simulink model "kinematics_model"  (R2023a)
settings: Solver=FixedStepAuto  StartTime=0.0  StopTime=fs  FixedStep=ts  RelTol=1e-3
undefined symbols (not defined in the file): alpha, eta_0, K_p, k_R, k_theta, p_0, theta_d, umax, umin, y_d
libraries: simulink_extras x1, slctrlblks x1, simulink x1
settings Model: Creator=mori_keigo  LastModifiedBy=mori_keigo

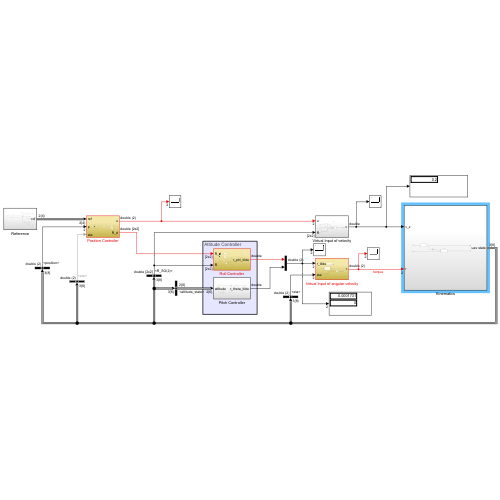
[thumbnail: Simulink's stored preview of the top-level diagram]
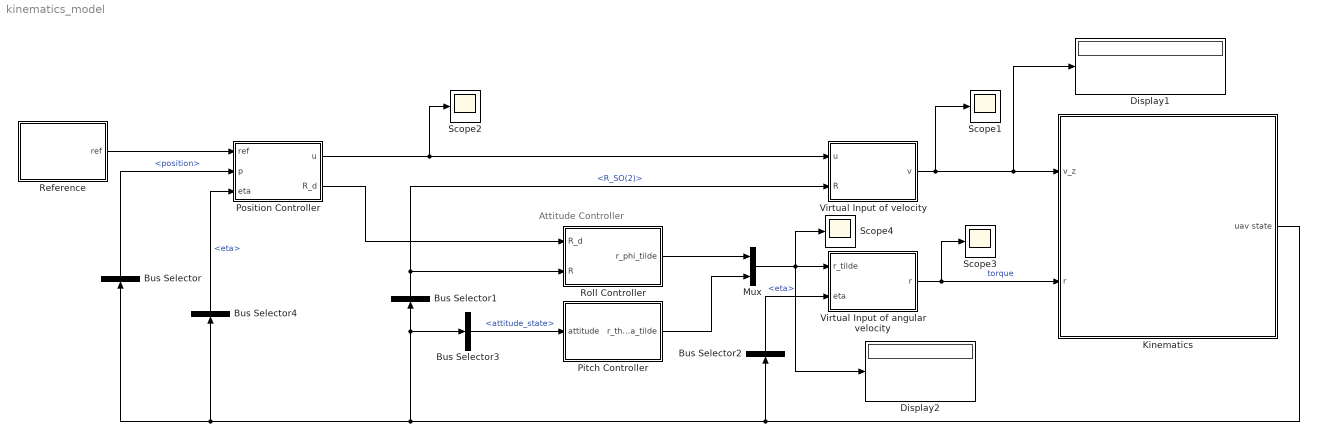
== system kinematics_model ==
  note: Attitude Controller
  Bus Selector : BusSelector  OutputSignals=translation_state.position
  Bus Selector1 : BusSelector  OutputSignals=attitude_state.R_SO(2)
  Bus Selector2 : BusSelector  OutputSignals=attitude_state.eta
  Bus Selector3 : BusSelector  OutputSignals=attitude_state
  Bus Selector4 : BusSelector  OutputSignals=attitude_state.eta
  Display1 : Display
  Display2 : Display
  Kinematics : Subsystem
  Mux : Mux  Inputs=2
  Pitch Controller : Subsystem
  Position Controller : Subsystem
  Reference : Subsystem
  Roll Controller : Subsystem
  Scope{1..4} (4 alike) : Scope
  Virtual Input of angular velocity : Subsystem
  Virtual Input of velocity : Subsystem
  wires:
  Bus Selector/1 -> Position Controller/2(p)  "<position>"
  Reference/1(ref) -> Position Controller/1(ref)
  Position Controller/2(R_d) -> Roll Controller/1(R_d)
  Kinematics/1(uav state) -> Bus Selector/1, Bus Selector4/1, Bus Selector1/1, Bus Selector3/1, Bus Selector2/1
  Virtual Input of velocity/1(v) -> Display1/1, Kinematics/1(v_z), Scope1/1
  Roll Controller/1(r_phi_tilde) -> Mux/1
  Pitch Controller/1(r_theta_tilde) -> Mux/2
  Mux/1 -> Scope4/1, Display2/1, Virtual Input of angular velocity/1(r_tilde)
  Bus Selector3/1 -> Pitch Controller/1(attitude)  "<attitude_state>"
  Bus Selector1/1 -> Roll Controller/2(R), Virtual Input of velocity/2(R)  "<R_SO(2)>"
  Bus Selector2/1 -> Virtual Input of angular velocity/2(eta)  "<eta>"
  Position Controller/1(u) -> Scope2/1, Virtual Input of velocity/1(u)
  Bus Selector4/1 -> Position Controller/3(eta)  "<eta>"
  Virtual Input of angular velocity/1(r) -> Kinematics/2(r), Scope3/1  "torque"

== system kinematics_model/Kinematics ==
  note: $\dot{\eta} = A r$
  note: $\dot{p} = Rv$
  v_z : Inport
  r : Inport  Port=2
  Bus Selector : BusSelector  OutputSignals=eta
  Kinematics of Attitude : Subsystem
  Kinematics of Translation : Subsystem
  Out Bus Element : Outport  PortName=uav state  Element=attitude_state
  Out Bus Element1 : Outport  PortName=uav state  Element=translation_state
  wires:
  r/1 -> Kinematics of Attitude/1(r)
  Kinematics of Translation/1(uav state) -> Out Bus Element1/1  "translation_state"
  v_z/1 -> Kinematics of Translation/2(v_z)  "attitude_state"
  Kinematics of Attitude/1(attitude_state) -> Bus Selector/1, Out Bus Element/1
  Bus Selector/1 -> Kinematics of Translation/1(eta)  "<eta>"

== system kinematics_model/Pitch Controller ==
  note: $\tilde{r}_{\theta} = k_{\theta} (\theta_d - \theta)$
  attitude : Inport
  Bus Selector : BusSelector  OutputSignals=eta
  Gain : Gain  Gain=k_theta
  Selector : Selector  InputPortWidth=2  IndexOptions=Index vector (dialog)  Indices=[2]  OutputSizes=1
  Sum : Sum  Inputs=|+-
  theta_d : Constant  Value=theta_d
  r_theta_tilde : Outport
  wires:
  attitude/1 -> Bus Selector/1
  theta_d/1 -> Sum/1
  Sum/1 -> Gain/1
  Gain/1 -> r_theta_tilde/1
  Bus Selector/1 -> Selector/1  "<eta>"
  Selector/1 -> Sum/2

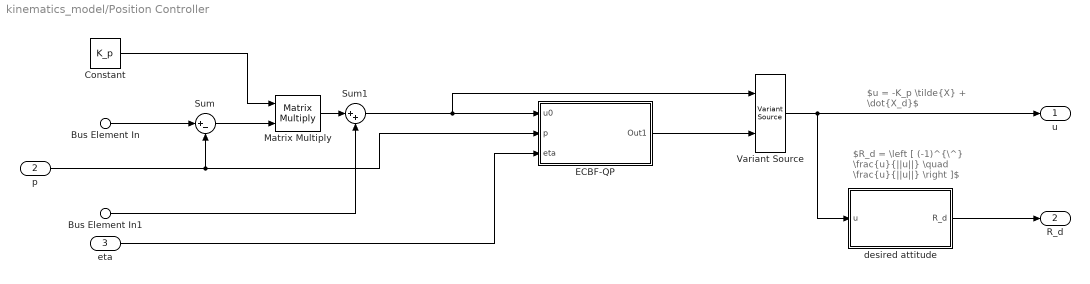
== system kinematics_model/Position Controller ==
  note: $u = -K_p \tilde{X} + \dot{X_d}$
  note: $R_d = \left [ (-1)^{\^} \frac{u}{||u||} \quad \frac{u}{||u||} \right ]$
  Bus Element In : Inport  PortName=ref  Element=p_d
  Bus Element In1 : Inport  PortName=ref  Element=p_d_dot
  p : Inport  Port=2
  eta : Inport  Port=3
  Constant : Constant  Value=K_p
  ECBF-QP : Subsystem
  Matrix Multiply : Product  Multiplication=Matrix(*)
  Sum : Sum  Inputs=|+-
  Sum1 : Sum  Inputs=|++
  Variant Source : VariantSource
  desired attitude : Subsystem
  u : Outport
  R_d : Outport  Port=2
  wires:
  Bus Element In/1 -> Sum/1
  Bus Element In1/1 -> Sum1/2
  desired attitude/1(R_d) -> R_d/1
  Matrix Multiply/1 -> Sum1/1
  Constant/1 -> Matrix Multiply/1
  Sum/1 -> Matrix Multiply/2
  Sum1/1 -> Variant Source/1, ECBF-QP/1(u0)
  ECBF-QP/1(Out1) -> Variant Source/2
  eta/1 -> ECBF-QP/3(eta)
  Variant Source/1 -> desired attitude/1(u), u/1
  p/1 -> ECBF-QP/2(p), Sum/2

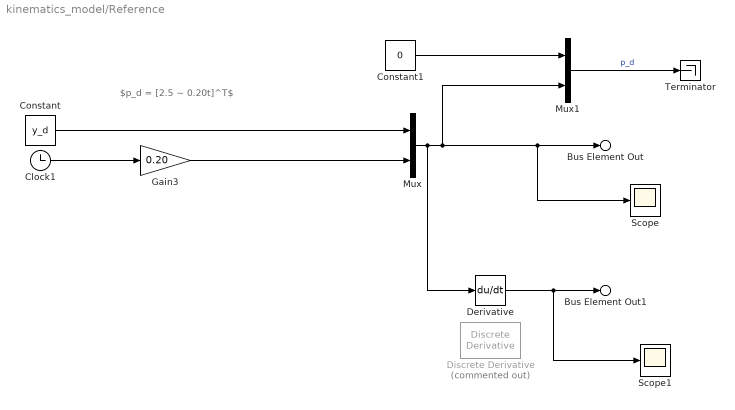
== system kinematics_model/Reference ==
  note: $p_d = [2.5 ~ 0.20t]^T$
  Clock1 : Clock
  Constant : Constant  Value=y_d
  Constant1 : Constant  Value=0
  Derivative : Derivative
  Discrete Derivative : simulink/Discrete/Discrete Derivative  Commented=on  gainval=1.0  ICPrevScaledInput=0.0  OutMin=[]  OutMax=[]  OutDataType=fixdt(1, 16)  OutScaling=2^-10  DoSatur=off
  Gain3 : Gain  Gain=0.20
  Mux : Mux  Inputs=2
  Mux1 : Mux  Inputs=2
  Scope : Scope
  Scope1 : Scope
  Terminator : Terminator
  Bus Element Out : Outport  PortName=ref  Element=p_d
  Bus Element Out1 : Outport  PortName=ref  Element=p_d_dot
  wires:
  Derivative/1 -> Scope1/1, Bus Element Out1/1
  Clock1/1 -> Gain3/1
  Gain3/1 -> Mux/2
  Mux/1 -> Mux1/2, Scope/1, Bus Element Out/1, Derivative/1
  Constant1/1 -> Mux1/1
  Mux1/1 -> Terminator/1  "p_d"
  Constant/1 -> Mux/1

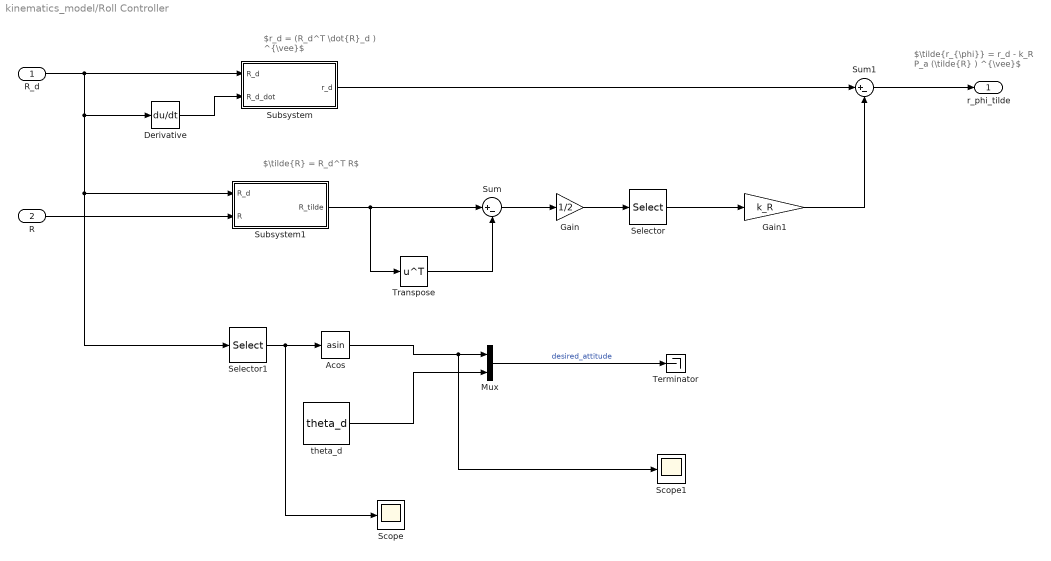
== system kinematics_model/Roll Controller ==
  note: $r_d = (R_d^T \dot{R}_d ) ^{\vee}$
  note: $\tilde{r_{\phi}} = r_d - k_R P_a (\tilde{R} ) ^{\vee}$
  note: $\tilde{R} = R_d^T R$
  R_d : Inport
  R : Inport  Port=2
  Acos : Trigonometry  Operator=asin
  Derivative : Derivative
  Gain : Gain  Gain=1/2
  Gain1 : Gain  Gain=k_R
  Mux : Mux  Inputs=2
  Scope : Scope
  Scope1 : Scope
  Selector : Selector  NumberOfDimensions=2  InputPortWidth=3  IndexOptions=Index vector (dialog),Index vector (dialog)  Indices=[2],1  OutputSizes=1,1
  Selector1 : Selector  NumberOfDimensions=2  InputPortWidth=3  IndexOptions=Index vector (dialog),Index vector (dialog)  Indices=[2],[1]  OutputSizes=1,1
  Subsystem : Subsystem
  Subsystem1 : Subsystem
  Sum : Sum  Inputs=|+-
  Sum1 : Sum  Inputs=|+-
  Terminator : Terminator
  Transpose : Math  Operator=transpose
  theta_d : Constant  Value=theta_d
  r_phi_tilde : Outport
  wires:
  Derivative/1 -> Subsystem/2(R_d_dot)
  Subsystem1/1(R_tilde) -> Transpose/1, Sum/1
  Transpose/1 -> Sum/2
  Sum/1 -> Gain/1
  Gain/1 -> Selector/1
  Selector/1 -> Gain1/1
  Sum1/1 -> r_phi_tilde/1
  Subsystem/1(r_d) -> Sum1/1
  Gain1/1 -> Sum1/2
  R_d/1 -> Selector1/1, Subsystem1/1(R_d), Derivative/1, Subsystem/1(R_d)
  Selector1/1 -> Scope/1, Acos/1
  R/1 -> Subsystem1/2(R)
  Acos/1 -> Scope1/1, Mux/1
  theta_d/1 -> Mux/2
  Mux/1 -> Terminator/1  "desired_attitude"

== system kinematics_model/Virtual Input of angular velocity ==
  note: $r = A^{-1} \tilde{r}$
  r_tilde : Inport
  eta : Inport  Port=2
  Product : Product  Inputs=/*  Multiplication=Matrix(*)
  Transformation to A : Subsystem
  r : Outport
  wires:
  Transformation to A/1(A) -> Product/1
  r_tilde/1 -> Product/2
  Product/1 -> r/1
  eta/1 -> Transformation to A/1(eta)

== system kinematics_model/Virtual Input of velocity ==
  note: $v_z = u^T Re_2$
  u : Inport
  R : Inport  Port=2
  Constant : Constant  Value=[0;1]  VectorParams1D=off
  Matrix Multiply : Product  Inputs=3  Multiplication=Matrix(*)
  Transpose : Math  Operator=transpose
  v : Outport
  wires:
  R/1 -> Matrix Multiply/2
  Transpose/1 -> Matrix Multiply/1
  Matrix Multiply/1 -> v/1
  u/1 -> Transpose/1
  Constant/1 -> Matrix Multiply/3

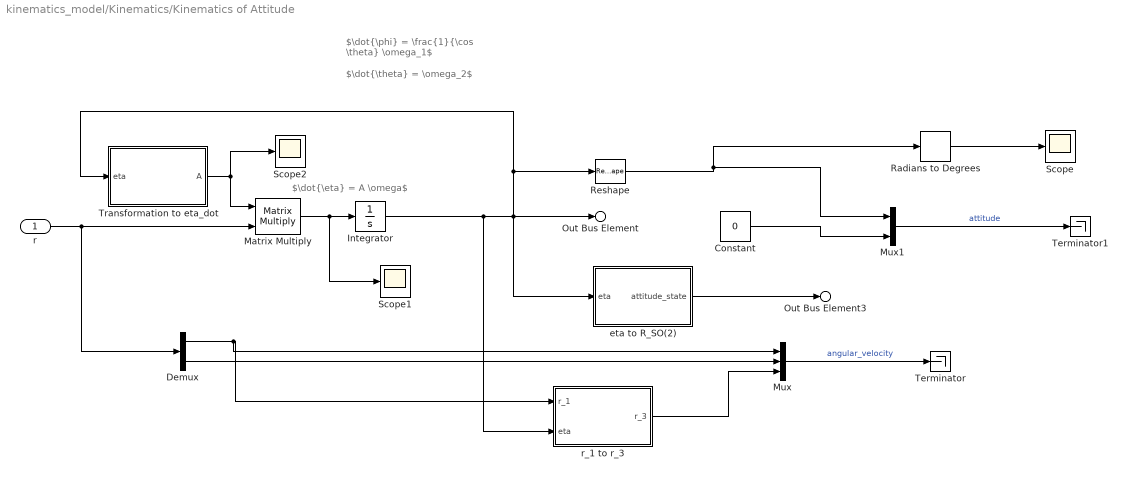
== system kinematics_model/Kinematics/Kinematics of Attitude ==
  note: $\dot{\theta} = \omega_2$
  note: $\dot{\phi} = \frac{1}{\cos \theta} \omega_1$
  note: $\dot{\eta} = A \omega$
  r : Inport
  Constant : Constant  Value=0
  Demux : Demux  Outputs=2
  Integrator : Integrator  InitialCondition=eta_0
  Matrix Multiply : Product  Multiplication=Matrix(*)
  Mux : Mux  Inputs=3
  Mux1 : Mux  Inputs=2
  Radians to Degrees : simulink_extras/Transformations/Radians to Degrees
  Reshape : Reshape
  Scope : Scope
  Scope1 : Scope
  Scope2 : Scope
  Terminator : Terminator
  Terminator1 : Terminator
  Transformation to eta_dot : Subsystem
  eta to R_SO(2) : Subsystem
  r_1 to r_3 : Subsystem
  Out Bus Element : Outport  PortName=attitude_state  Element=eta
  Out Bus Element3 : Outport  PortName=attitude_state  Element=R_SO(2)
  wires:
  Integrator/1 -> r_1 to r_3/2(eta), Out Bus Element/1, eta to R_SO(2)/1(eta), Transformation to eta_dot/1(eta), Reshape/1
  Matrix Multiply/1 -> Scope1/1, Integrator/1
  r/1 -> Demux/1, Matrix Multiply/2
  Transformation to eta_dot/1(A) -> Matrix Multiply/1, Scope2/1
  eta to R_SO(2)/1(attitude_state) -> Out Bus Element3/1
  Demux/1 -> Mux/1, r_1 to r_3/1(r_1)
  r_1 to r_3/1(r_3) -> Mux/3
  Demux/2 -> Mux/2
  Mux/1 -> Terminator/1  "angular_velocity"
  Radians to Degrees/1 -> Scope/1
  Reshape/1 -> Mux1/1, Radians to Degrees/1
  Constant/1 -> Mux1/2
  Mux1/1 -> Terminator1/1  "attitude"

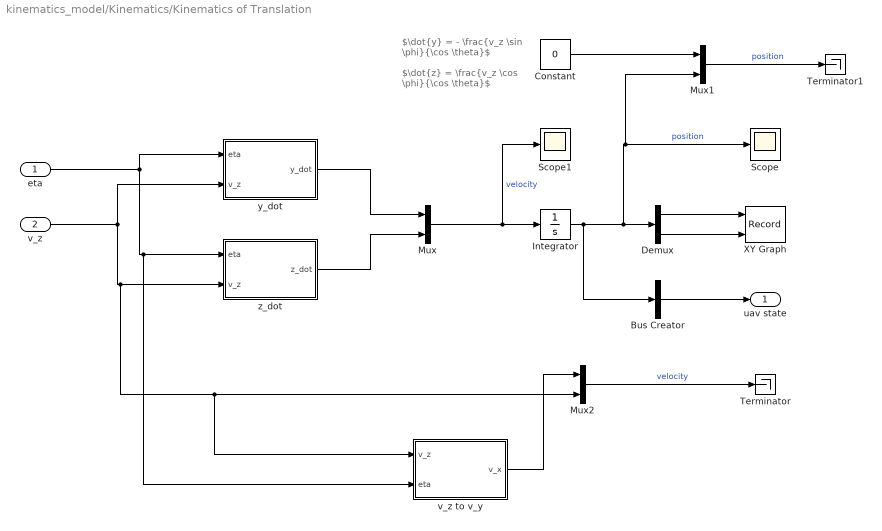
== system kinematics_model/Kinematics/Kinematics of Translation ==
  note: $\dot{z} = \frac{v_z \cos \phi}{\cos \theta}$
  note: $\dot{y} = - \frac{v_z \sin \phi}{\cos \theta}$
  eta : Inport
  v_z : Inport  Port=2
  Bus Creator : BusCreator  Inputs=1
  Constant : Constant  Value=0
  Demux : Demux  Outputs=2
  Integrator : Integrator  InitialCondition=p_0
  Mux : Mux  Inputs=2
  Mux1 : Mux  Inputs=2
  Mux2 : Mux  Inputs=2
  Scope : Scope
  Scope1 : Scope
  Terminator : Terminator
  Terminator1 : Terminator
  XY Graph : Record  FileSettingsInternal="{\"entries\":[{\"content\":{\"excelSettings\":{\"content\":{},\"type\":\"Streamout.ExcelSettings\"}},\"type\":\"Streamout.FileSettingStorage\",\"uuid\":\"\"}],\"packageUris\":[\"http:\\/\\/schema.mathworks.com\\/mf0\\/streamout_blocks\\/R2020a\"],\"version\":\"1.0\"}"  Layout=[1 1]  SignalsInternal="{\"entries\":[{\"content\":{\"signals\":[{\"content\":{\"blockPath\":[],\"dimensions\":[1],\"domain\":\"\",\"lineColor\":\"#a2142f\",\"plots\":[1],\"port\":1,\"sid\":[\"\"],\"signalID\":39,\"signalName\":\"Demux:1\"},\"type\":\"RecordBlkView.Signal\",\"uuid\":\"\"},{\"content\":{\"blockPath\":[],\"dimensions\":[1],\"domain\":\"\",\"lineColor\":\"#139fff\",\"plots\":[1],\"port\":2,\"sid\":[\"\"],\"signalID\":43,\"signalName\":\"Demux:2\"},\"type\":\"RecordBlkView.Signal\",\"uuid\":\"\"}]},\"type\":\"RecordBlkView.InputSignals\",\"uuid\":\"\"}],\"packageUris\":[\"http:\\/\\/schema.mathworks.com\\/mf0\\/streamout_blocks\\/R2020a\"],\"version\":\"1.0\"}"  VisualizationBindings="{\"xyplotplugin\":{\"info\":[{\"series\":[{\"bindingParametersList\":[{\"parameter\":\"X-Axis\",\"signalID\":39,\"signalName\":\"Demux:1\"},{\"parameter\":\"Y-Axis\",\"signalID\":43,\"signalName\":\"Demux:2\"}],\"seriesID\":24023}],\"subplotID\":1}]}}"  CompatibilityTag=XY
  v_z to v_y : Subsystem
  y_dot : Subsystem
  z_dot : Subsystem
  uav state : Outport
  wires:
  Integrator/1 -> Mux1/2, Scope/1, Demux/1, Bus Creator/1  "position"
  Mux/1 -> Scope1/1, Integrator/1  "velocity"
  Bus Creator/1 -> uav state/1
  eta/1 -> v_z to v_y/2(eta), z_dot/1(eta), y_dot/1(eta)
  y_dot/1(y_dot) -> Mux/1
  v_z/1 -> v_z to v_y/1(v_z), Mux2/2, z_dot/2(v_z), y_dot/2(v_z)
  z_dot/1(z_dot) -> Mux/2
  Demux/1 -> XY Graph/1
  Demux/2 -> XY Graph/2
  Mux2/1 -> Terminator/1  "velocity"
  v_z to v_y/1(v_x) -> Mux2/1
  Constant/1 -> Mux1/1
  Mux1/1 -> Terminator1/1  "position"

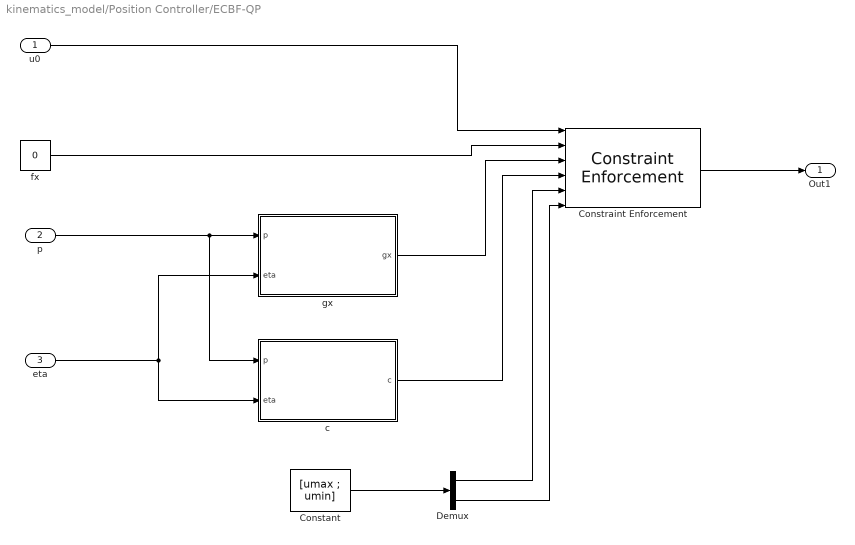
== system kinematics_model/Position Controller/ECBF-QP ==
  u0 : Inport
  p : Inport  Port=2
  eta : Inport  Port=3
  Constant : Constant  Value=[umax ; umin]  VectorParams1D=off
  Constraint Enforcement : slctrlblks/Constraint Enforcement  nc=1  nu=2  c=0  external_c=on  external_umax=on  external_umin=on  Ts=0.01  maxiter=200  tol=1e-6  output_exitflag=off  relax_c=off  relax_u=off
  Demux : Demux  Outputs=2
  c : Subsystem
  fx : Constant  Value=0  VectorParams1D=off
  gx : Subsystem
  Out1 : Outport
  wires:
  u0/1 -> Constraint Enforcement/1
  p/1 -> c/1(p), gx/1(p)
  eta/1 -> gx/2(eta), c/2(eta)
  fx/1 -> Constraint Enforcement/2
  gx/1(gx) -> Constraint Enforcement/3
  c/1(c) -> Constraint Enforcement/4
  Constraint Enforcement/1 -> Out1/1
  Constant/1 -> Demux/1
  Demux/1 -> Constraint Enforcement/5
  Demux/2 -> Constraint Enforcement/6

== system kinematics_model/Position Controller/desired attitude ==
  u : Inport
  (-1)^ : Constant  Value=[0 1; -1 0]  VectorParams1D=off
  Divide : Product  Inputs=*/
  Dot Product : DotProduct  OutDataTypeStr=Inherit: Inherit via internal rule
  Matrix Concatenate : Concatenate  Mode=Multidimensional array  ConcatenateDimension=2
  Matrix Multiply : Product  Multiplication=Matrix(*)
  Square Root : Sqrt
  R_d : Outport
  wires:
  Dot Product/1 -> Square Root/1
  u/1 -> Divide/1, Dot Product/2, Dot Product/1
  Square Root/1 -> Divide/2
  Matrix Concatenate/1 -> R_d/1
  Divide/1 -> Matrix Concatenate/2, Matrix Multiply/2
  (-1)^/1 -> Matrix Multiply/1
  Matrix Multiply/1 -> Matrix Concatenate/1

== system kinematics_model/Roll Controller/Subsystem ==
  R_d : Inport
  R_d_dot : Inport  Port=2
  Matrix Multiply : Product  Multiplication=Matrix(*)
  Selector : Selector  NumberOfDimensions=2  InputPortWidth=3  IndexOptions=Index vector (dialog),Index vector (dialog)  Indices=[2],1  OutputSizes=1,1
  Transpose : Math  Operator=transpose
  r_d : Outport
  wires:
  R_d/1 -> Transpose/1
  Transpose/1 -> Matrix Multiply/1
  R_d_dot/1 -> Matrix Multiply/2
  Matrix Multiply/1 -> Selector/1
  Selector/1 -> r_d/1

== system kinematics_model/Roll Controller/Subsystem1 ==
  R_d : Inport
  R : Inport  Port=2
  Matrix Multiply : Product  Multiplication=Matrix(*)
  Transpose : Math  Operator=transpose
  R_tilde : Outport
  wires:
  R_d/1 -> Transpose/1
  Transpose/1 -> Matrix Multiply/1
  R/1 -> Matrix Multiply/2
  Matrix Multiply/1 -> R_tilde/1

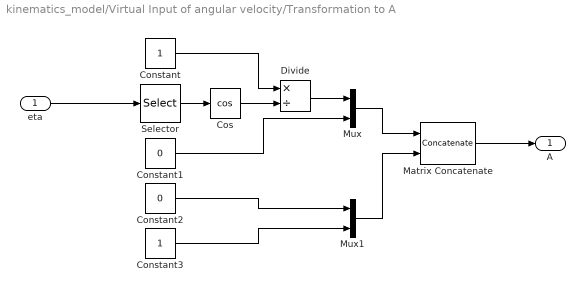
== system kinematics_model/Virtual Input of angular velocity/Transformation to A ==
  eta : Inport
  Constant : Constant
  Constant1 : Constant  Value=0
  Constant2 : Constant  Value=0
  Constant3 : Constant
  Cos : Trigonometry  Operator=cos
  Divide : Product  Inputs=*/
  Matrix Concatenate : Concatenate  Mode=Multidimensional array  ConcatenateDimension=2
  Mux : Mux  Inputs=2
  Mux1 : Mux  Inputs=2
  Selector : Selector  InputPortWidth=2  IndexOptions=Index vector (dialog)  Indices=[2]  OutputSizes=1
  A : Outport
  wires:
  eta/1 -> Selector/1
  Constant/1 -> Divide/1
  Divide/1 -> Mux/1
  Constant1/1 -> Mux/2
  Constant2/1 -> Mux1/1
  Constant3/1 -> Mux1/2
  Mux/1 -> Matrix Concatenate/1
  Mux1/1 -> Matrix Concatenate/2
  Matrix Concatenate/1 -> A/1
  Selector/1 -> Cos/1
  Cos/1 -> Divide/2

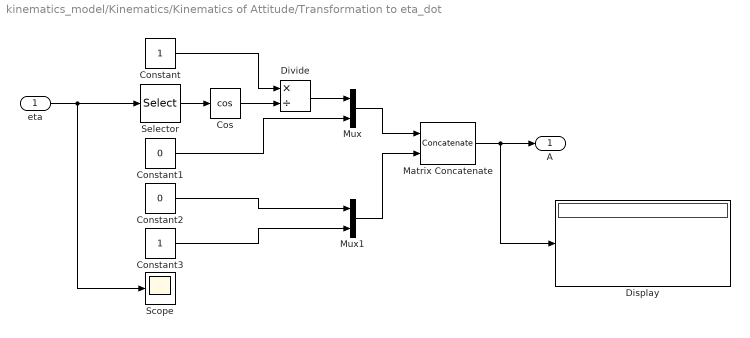
== system kinematics_model/Kinematics/Kinematics of Attitude/Transformation to eta_dot ==
  eta : Inport
  Constant : Constant
  Constant1 : Constant  Value=0
  Constant2 : Constant  Value=0
  Constant3 : Constant
  Cos : Trigonometry  Operator=cos
  Display : Display
  Divide : Product  Inputs=*/
  Matrix Concatenate : Concatenate  Mode=Multidimensional array  ConcatenateDimension=2
  Mux : Mux  Inputs=2
  Mux1 : Mux  Inputs=2
  Scope : Scope
  Selector : Selector  InputPortWidth=2  IndexOptions=Index vector (dialog)  Indices=[2]  OutputSizes=1
  A : Outport
  wires:
  eta/1 -> Scope/1, Selector/1
  Constant/1 -> Divide/1
  Divide/1 -> Mux/1
  Constant1/1 -> Mux/2
  Constant2/1 -> Mux1/1
  Constant3/1 -> Mux1/2
  Mux/1 -> Matrix Concatenate/1
  Mux1/1 -> Matrix Concatenate/2
  Matrix Concatenate/1 -> Display/1, A/1
  Selector/1 -> Cos/1
  Cos/1 -> Divide/2

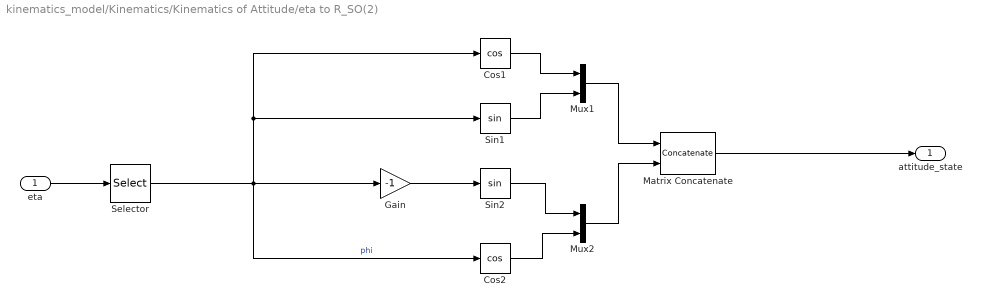
== system kinematics_model/Kinematics/Kinematics of Attitude/eta to R_SO(2) ==
  eta : Inport
  Cos1 : Trigonometry  Operator=cos
  Cos2 : Trigonometry  Operator=cos
  Gain : Gain  Gain=-1
  Matrix Concatenate : Concatenate  Mode=Multidimensional array  ConcatenateDimension=2
  Mux1 : Mux  Inputs=2
  Mux2 : Mux  Inputs=2
  Selector : Selector  InputPortWidth=2  IndexOptions=Index vector (dialog)  Indices=[1]  OutputSizes=1
  Sin1 : Trigonometry
  Sin2 : Trigonometry
  attitude_state : Outport
  wires:
  eta/1 -> Selector/1
  Cos2/1 -> Mux2/2
  Matrix Concatenate/1 -> attitude_state/1
  Mux2/1 -> Matrix Concatenate/2
  Mux1/1 -> Matrix Concatenate/1
  Gain/1 -> Sin2/1
  Cos1/1 -> Mux1/1
  Sin2/1 -> Mux2/1
  Sin1/1 -> Mux1/2
  Selector/1 -> Cos2/1, Gain/1, Cos1/1, Sin1/1  "phi"

== system kinematics_model/Kinematics/Kinematics of Attitude/r_1 to r_3 ==
  r_1 : Inport
  eta : Inport  Port=2
  Cos : Trigonometry  Operator=cos
  Divide : Product  Inputs=**/
  Gain : Gain  Gain=-1
  Selector : Selector  InputPortWidth=2  IndexOptions=Index vector (dialog)  Indices=[2]  OutputSizes=1
  Sin : Trigonometry
  r_3 : Outport
  wires:
  eta/1 -> Selector/1
  Selector/1 -> Cos/1, Sin/1
  r_1/1 -> Divide/1
  Sin/1 -> Divide/2
  Cos/1 -> Divide/3
  Divide/1 -> Gain/1
  Gain/1 -> r_3/1

== system kinematics_model/Kinematics/Kinematics of Translation/v_z to v_y ==
  v_z : Inport
  eta : Inport  Port=2
  Cos : Trigonometry  Operator=cos
  Divide : Product  Inputs=**/
  Gain : Gain  Gain=-1
  Selector : Selector  InputPortWidth=2  IndexOptions=Index vector (dialog)  Indices=[2]  OutputSizes=1
  Sin : Trigonometry
  v_x : Outport
  wires:
  v_z/1 -> Divide/1
  eta/1 -> Selector/1
  Selector/1 -> Cos/1, Sin/1
  Sin/1 -> Divide/2
  Cos/1 -> Divide/3
  Gain/1 -> v_x/1
  Divide/1 -> Gain/1

== system kinematics_model/Kinematics/Kinematics of Translation/y_dot ==
  eta : Inport
  v_z : Inport  Port=2
  Cos : Trigonometry  Operator=cos
  Demux : Demux  Outputs=2
  Divide : Product  Inputs=**/
  Gain1 : Gain  Gain=-1
  Sin1 : Trigonometry
  y_dot : Outport
  wires:
  Demux/1 -> Sin1/1
  Sin1/1 -> Divide/2
  v_z/1 -> Divide/1
  Demux/2 -> Cos/1
  Cos/1 -> Divide/3
  eta/1 -> Demux/1
  Gain1/1 -> y_dot/1
  Divide/1 -> Gain1/1

== system kinematics_model/Kinematics/Kinematics of Translation/z_dot ==
  eta : Inport
  v_z : Inport  Port=2
  Cos1 : Trigonometry  Operator=cos
  Cos2 : Trigonometry  Operator=cos
  Demux : Demux  Outputs=2
  Divide : Product  Inputs=**/
  z_dot : Outport
  wires:
  eta/1 -> Demux/1
  Demux/1 -> Cos2/1
  Demux/2 -> Cos1/1
  v_z/1 -> Divide/1
  Cos2/1 -> Divide/2
  Cos1/1 -> Divide/3
  Divide/1 -> z_dot/1

== system kinematics_model/Position Controller/ECBF-QP/c ==
  p : Inport
  eta : Inport  Port=2
  Cos : Trigonometry  Operator=cos
  Gain : Gain  Gain=alpha/2
  Product : Product
  Selector : Selector  InputPortWidth=2  IndexOptions=Index vector (dialog)  Indices=[2]  OutputSizes=1
  h : Subsystem
  c : Outport
  wires:
  eta/1 -> Selector/1
  p/1 -> h/1(p)
  Selector/1 -> Cos/1
  h/1(h) -> Gain/1
  Gain/1 -> Product/1
  Cos/1 -> Product/2
  Product/1 -> c/1

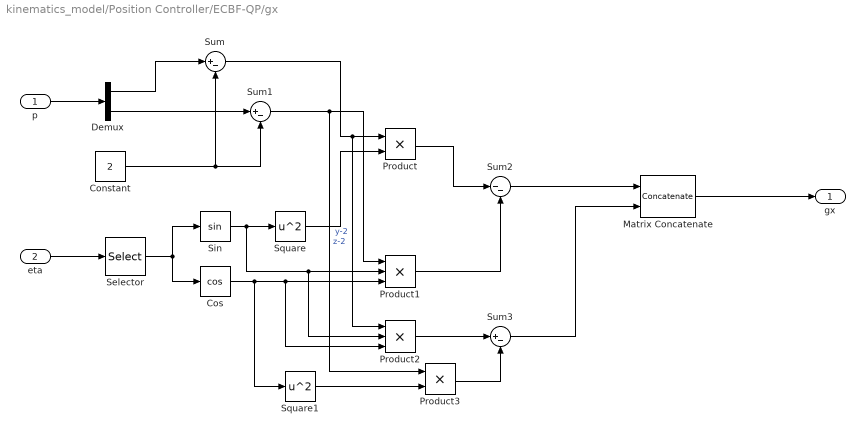
== system kinematics_model/Position Controller/ECBF-QP/gx ==
  p : Inport
  eta : Inport  Port=2
  Constant : Constant  Value=2
  Cos : Trigonometry  Operator=cos
  Demux : Demux  Outputs=2
  Matrix Concatenate : Concatenate  Mode=Multidimensional array  ConcatenateDimension=2
  Product : Product
  Product1 : Product  Inputs=3
  Product2 : Product  Inputs=3
  Product3 : Product
  Selector : Selector  InputPortWidth=2  IndexOptions=Index vector (dialog)  Indices=[1]  OutputSizes=1
  Sin : Trigonometry
  Square : Math  Operator=square
  Square1 : Math  Operator=square
  Sum : Sum  Inputs=|+-
  Sum1 : Sum  Inputs=|+-
  Sum2 : Sum  Inputs=|--
  Sum3 : Sum  Inputs=|+-
  gx : Outport
  wires:
  p/1 -> Demux/1
  Demux/1 -> Sum/1
  Constant/1 -> Sum1/2, Sum/2
  Demux/2 -> Sum1/1
  eta/1 -> Selector/1
  Selector/1 -> Sin/1, Cos/1
  Sin/1 -> Product2/2, Product1/2, Square/1
  Square/1 -> Product/2
  Sum/1 -> Product2/1, Product/1  "y-2"
  Product/1 -> Sum2/1
  Cos/1 -> Square1/1, Product2/3, Product1/3
  Sum1/1 -> Product3/1, Product1/1  "z-2"
  Product1/1 -> Sum2/2
  Sum2/1 -> Matrix Concatenate/1
  Matrix Concatenate/1 -> gx/1
  Product2/1 -> Sum3/1
  Square1/1 -> Product3/2
  Sum3/1 -> Matrix Concatenate/2
  Product3/1 -> Sum3/2

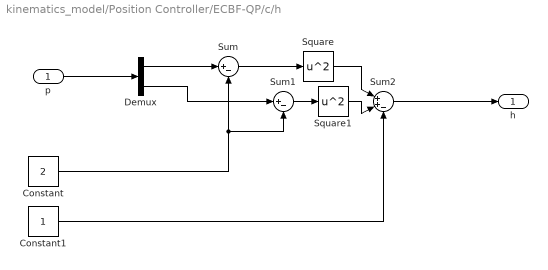
== system kinematics_model/Position Controller/ECBF-QP/c/h ==
  p : Inport
  Constant : Constant  Value=2
  Constant1 : Constant
  Demux : Demux  Outputs=2
  Square : Math  Operator=square
  Square1 : Math  Operator=square
  Sum : Sum  Inputs=|+-
  Sum1 : Sum  Inputs=|+-
  Sum2 : Sum  Inputs=|++-
  h : Outport
  wires:
  p/1 -> Demux/1
  Demux/1 -> Sum/1
  Constant/1 -> Sum1/2, Sum/2
  Demux/2 -> Sum1/1
  Constant1/1 -> Sum2/3
  Sum2/1 -> h/1
  Sum/1 -> Square/1
  Sum1/1 -> Square1/1
  Square/1 -> Sum2/1
  Square1/1 -> Sum2/2
